simulink model "wheelmodsimscape"  (R2023a)
settings: Solver=ode23t  StartTime=0.0  StopTime=20  RelTol=1e-3
values from neighbouring files (symbols this model uses):
  angleT = 0    [rovervars.mat]    (also in varedit.m)
  mass = 1    [rovervars.mat]    (also in varedit.m)
  massRover = 50    [rovervars.mat]    (also in varedit.m)
  pwmVolt = 5    [rovervars.mat]    (also in varedit.m)
  radius = 0.1    [rovervars.mat]    (also in varedit.m)
  rotorInertia = 200    [rovervars.mat]    (also in varedit.m)
libraries: ee_lib x24, fl_lib x18, sdl_lib x13, nesl_utility x6, SignalEditorBlockLib x1
settings Model: Creator=MY DELL  LastModifiedBy=MY DELL

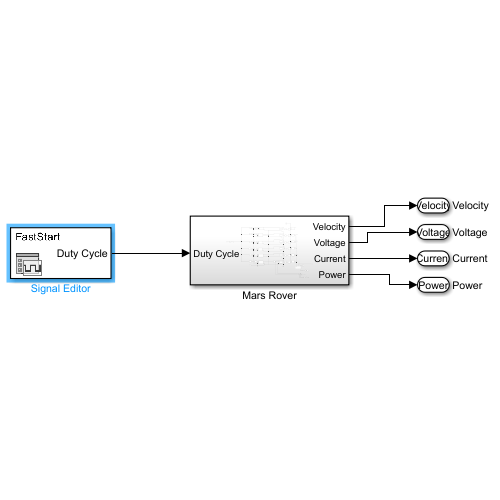
[thumbnail: Simulink's stored preview of the top-level diagram]
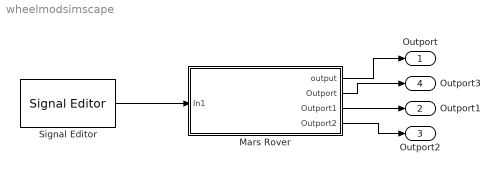
== system wheelmodsimscape ==
  Mars Rover : Subsystem
  Signal Editor : SignalEditorBlockLib/Signal Editor  FileName=signalscenario.mat  ActiveScenario=FastStart  ActiveSignal=Duty Cycle  IsBus=off  OutputBusObjectStr=Bus: BusObject  SampleTime=0  ZeroCross=off  OutputAfterFinalValue=Setting to zero  Unit=inherit  PreserveSignalName=on  ApplySigPropsToAllScenarios=on
  Outport : Outport  SignalName=Velocity
  Outport1 : Outport  Port=2  SignalName=Current
  Outport2 : Outport  Port=3  SignalName=Power
  Outport3 : Outport  Port=4  SignalName=Voltage
  wires:
  Signal Editor/1 -> Mars Rover/1(In1)
  Mars Rover/1(output) -> Outport/1
  Mars Rover/2(Outport) -> Outport3/1
  Mars Rover/3(Outport1) -> Outport1/1
  Mars Rover/4(Outport2) -> Outport2/1

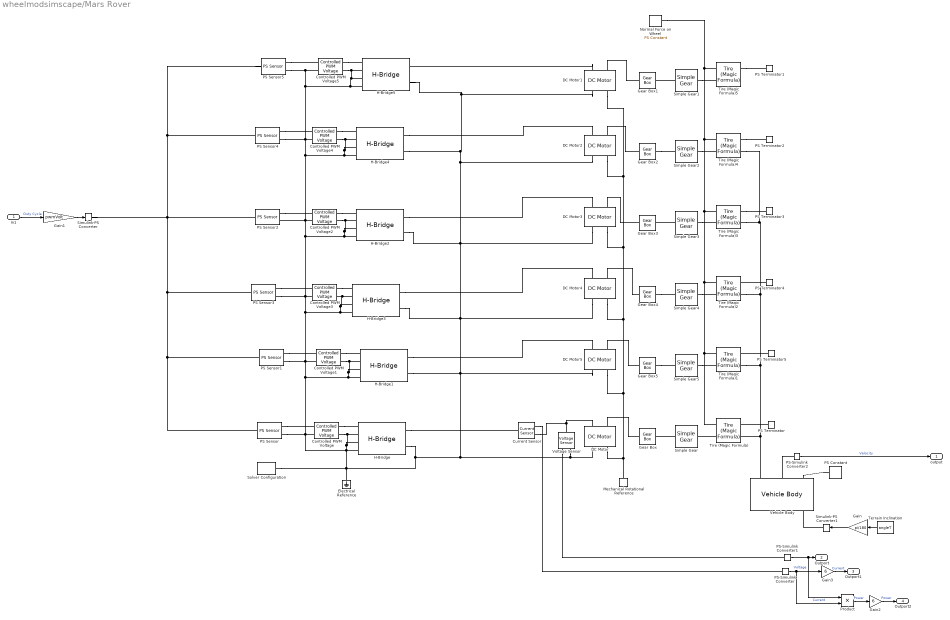
== system wheelmodsimscape/Mars Rover ==
  In1 : Inport
  Controlled PWM Voltage{,1..5} (6 alike) : ee_lib/Integrated Circuits/Controlled PWM Voltage  F=4000 Hz  TD=0 s  pulse_width_offset=0 s  pulse_min=0 s  pwm_or_av=ee.enum.pwm_or_av.averaged  event_type=ee.enum.ic.event.asynchronous  sample_time=1e-6 s  Vmin=0 V  Vmax=pwmVolt V  Vm=pwmVolt V  u_min=0  u_max=1
  Current Sensor : fl_lib/Electrical/Electrical Sensors/Current Sensor
  DC Motor{,1..5} (6 alike) : ee_lib/Electromechanical/Brushed Motors/DC Motor  field_option=ee.enum.field_option.pm  Rf=100 Ohm  Lf=1 H  Laf=0.15 H  If0=0 A  parameterization=ee.enum.dcparam_option.torque_speed  Ra=3.9 Ohm  La=inductance H  emf_or_torque=ee.enum.emf_or_torque.kv  Kv=0.072e-3 V/rpm  Ki=6.876e-4 N*m/A  T_stall=stallTorque N*m  w_max=noloadSpeed rpm  w_rated=15000 rpm  P_rated=0.08 W  V_rated=ratedVolt V  lam_param=ee.enum.lam_param.current  i_noload=noloadCurrent A  V_i_noload=ratedVolt V  J=rotorInertia cm^2*g  lam=0 N*m*s/rad  speed0=0 rpm  enable_fault_armature=simscape.enum.onoff.off  rev_faulted=1 / 3  G_faulted_armature=1e-5 S  fault_trigger_armature=ee.enum.faults.faultTrigger.temporal  t_fault_armature=1 s  max_permissible_current_armature=inf A  t_fail_on_current_armature=1 s  enable_fault_field=simscape.enum.onoff.off  G_faulted_field=1e-5 S  fault_trigger_field=ee.enum.faults.faultTrigger.temporal  t_fault_field=1 s  max_permissible_current_field=inf A  t_fail_on_current_field=1 s  fault_action=simscape.enum.assert.action.none  alpha=3.93e-3 1/K  Tmeas=25 degC  thermal_mass=100 J/K  initial_temperature=25 degC
  Electrical Reference : fl_lib/Electrical/Electrical Elements/Electrical Reference
  Gain : Gain  Gain=pi/180
  Gain1 : Gain  Gain=pwmVolt
  Gain2 : Gain  Gain=6
  Gain3 : Gain  Gain=6
  Gear Box{,1..5} (6 alike) : fl_lib/Mechanical/Mechanisms/Gear Box  ratio=100  t_in_specify=off  t_in_priority=None  t_in=0 N*m  t_in_nominal_specify=off  t_in_nominal_unit=N*m  t_in_nominal_value=1  t_out_specify=off  t_out_priority=None  t_out=0 N*m  t_out_nominal_specify=off  t_out_nominal_unit=N*m  t_out_nominal_value=1
  H-Bridge{,1..5} (6 alike) : ee_lib/Semiconductors & Converters/Converters/H-Bridge  supply_ports=ee.enum.supply_ports.hidesupply  pwm_or_av=ee.enum.pwm_or_av.averaged  regenerative_braking_mode=ee.enum.converters.regenerative_braking_mode.depends_on_rev  discontinuous=ee.enum.current_profile.continuous  freewheeling_mode=ee.enum.converters.freewheeling_mode.one_switch_one_diode  Rload=10 Ohm  Lload=1e-5 H  F=10 kHz  Venable=pwmVolt/2 V  Vmax=pwmVolt V  Vreverse=pwmVolt/2 V  Vbrake=pwmVolt/2 V  Vm=ratedVolt V  Ron=1e-6 Ohm  Don=0.05 Ohm  Goff=1e-6 S  Tmeas=298.15 K  Ron2=0.1 Ohm  Don2=0.05 Ohm  Tmeas2=398.15 K  thermal_mass=100 J/K  initial_temperature=298.15 K
  Mechanical Rotational Reference : fl_lib/Mechanical/Rotational Elements/Mechanical Rotational Reference
  Normal Force on Wheel : fl_lib/Physical Signals/Sources/PS Constant  constant=massRover*9.81/6 N
  PS Constant : fl_lib/Physical Signals/Sources/PS Constant  constant=windSpeed m/s
  PS Sensor{,1..5} (6 alike) : ee_lib/Sensors & Transducers/PS Sensor  op_type=1  A=1  B=0  Ymax=5  Ymin=0.01
      settings: InternalSimscapePortConfiguration="{\"Bottom\":[],\"Left\":[{\"id\":\"U\",\"label\":\"U\",\"type\":\"input\"}],\"Right\":[{\"id\":\"p\",\"label\":\"+\",\"type\":\"foundation.electrical.electrical\"},{\"id\":\"n\",\"label\":\"-\",\"type\":\"foundation.electrical.electrical\"}],\"Top\":[]}"
  PS Terminator{,1..5} (6 alike) : fl_lib/Physical Signals/Sinks/PS Terminator
  PS-Simulink Converter : nesl_utility/PS-Simulink Converter  PhysicalDomain=network_engine_domain  SubClassName=ps_output  LeftPortType=input  RightPortType=output  PseudoPeriodic=off  Frequencies=[]  VectorFormat=inherit  Unit=inherit  AffineConversion=off
  PS-Simulink Converter1 : nesl_utility/PS-Simulink Converter  PhysicalDomain=network_engine_domain  SubClassName=ps_output  LeftPortType=input  RightPortType=output  PseudoPeriodic=off  Frequencies=[]  VectorFormat=inherit  Unit=inherit  AffineConversion=off
  PS-Simulink Converter2 : nesl_utility/PS-Simulink Converter  PhysicalDomain=network_engine_domain  SubClassName=ps_output  LeftPortType=input  RightPortType=output  PseudoPeriodic=off  Frequencies=[]  VectorFormat=inherit  Unit=inherit  AffineConversion=off
  Product : Product
  Simple Gear{,1..5} (6 alike) : sdl_lib/Gears/Simple Gear  ratio=1  rotation_direction=sdl.enum.shaftOutputDirection.same  friction_model=sdl.enum.gear_efficiencies_load.constant  T_noload=0.1 N*m  T_nom=5 N*m  efficiency_nom=0.8  efficiency=0.8  temperature_TLU=[280, 300, 320] K  load_TLU=[1, 5, 10] N*m  efficiency_TLU=[.95, .9, .85]  efficiency_TLU2=[.85, .8, .75; .95, .9, .85; .85, .8, .7]  w_thr=0.01 rad/s  pwr_thr=0.001 W  enable_backlash=false  hardstop_model=simscape.enum.hardstop.smooth  backlash_distance=1e-3 mm  r_base=0.1 m  transition=1e-4 mm  backlash_stiffness=1e6 N/m  backlash_damping=1e3 N*s/m  coeff_rest=0.7  v_tol=0.001 m/s  f_tol=0.001 N  mu_visc=[0, 0] N*m*s/rad  enable_faults=simscape.enum.onoff.off  efficiency_fault=0.05  external_fault=simscape.enum.onoff.off  temporal_fault=simscape.enum.onoff.off  fault_time=5 s  fault_angles=pi / 12 rad  report_fault=simscape.enum.assert.action.none  thermal_mass=50 J/K  temperature_specify=off  temperature_priority=High  temperature=300 K  temperature_nominal_specify=off  temperature_nominal_unit=K  temperature_nominal_value=1  x_backlash_specify=off  x_backlash_priority=None  x_backlash=0 mm  x_backlash_nominal_specify=off  x_backlash_nominal_unit=mm  x_backlash_nominal_value=1  f_hardstop_specify=off  f_hardstop_priority=None  f_hardstop=0 N  f_hardstop_nominal_specify=off  f_hardstop_nominal_unit=N  f_hardstop_nominal_value=1  v_backlash_specify=off  v_backlash_priority=None  v_backlash=0 m/s  v_backlash_nominal_specify=off  v_backlash_nominal_unit=m/s  v_backlash_nominal_value=1
  Simulink-PS Converter : nesl_utility/Simulink-PS Converter  PhysicalDomain=network_engine_domain  SubClassName=ps_input  LeftPortType=input  RightPortType=output  PseudoPeriodic=off  Frequencies=[]  NoiseDistribution=none  NoiseParameters=[]  Unit=1  AffineConversion=off  FilteringAndDerivatives=provide  SimscapeFilterOrder=1  InputFilterTimeConstant=0.001  UdotUserProvided=0
  Simulink-PS Converter1 : nesl_utility/Simulink-PS Converter  PhysicalDomain=network_engine_domain  SubClassName=ps_input  LeftPortType=input  RightPortType=output  PseudoPeriodic=off  Frequencies=[]  NoiseDistribution=none  NoiseParameters=[]  Unit=1  AffineConversion=off  FilteringAndDerivatives=provide  SimscapeFilterOrder=1  InputFilterTimeConstant=0.001  UdotUserProvided=0
  Solver Configuration : nesl_utility/Solver Configuration  PhysicalDomain=network_engine_domain  SubClassName=solver  LeftPortType=input  RightPortType=generic  Tones=[]  Harmonics=[]  SimulateNoise=off  Profile=off  UseLocalSampling=off  EnableSwitchedLinearOptims=on  FrequencyDomain=off  UseCCode=off  RelTol=0.001  AbsTol=0.001  MinStep=1e-09  ToWorkspace=off  RevertToSquareIcSolve=off  NumHomotopyIterations=100  PhasorMode=off  PhasorModeNumHarmonics=1  ConsistencySolver=NEWTON_XTOL_AFTER_FTOL  IndexReductionMethod=DerivativeReplacement  DoDC=off  ResidualTolerance=1e-09  ConsistencyTolSource=GLOBAL  ConsistencyAbsTol=0.001  ConsistencyRelTol=0.001  ConsistencyTolFactor=0.001  UseLocalSolver=off  LocalSolverChoice=NE_BACKWARD_EULER_ADVANCER  ResolveIndetEquations=on  FunctionEvalNumThread=1  LocalSolverSampleTime=0.001  DoFixedCost=off  MaxNonlinIter=3  MaxModeIter=2  ComputeImpulses=off  ImpulseIterations=2  LinearAlgebra=auto  LinearAlgebraNumThread=0  EquationFormulation=NE_TIME_EF  DelaysMemoryBudget=1024  AutomaticFiltering=on  FilteringTimeConstant=0.001  PartitionStorageMethod=AS_NEEDED  PartitionMemoryBudget=1024  PartitionMethod=ROBUST
  Terrain Inclination : Constant  Value=angleT
  Tire (Magic Formula){,1..5} (6 alike) : sdl_lib/Tires & Vehicles/Tire (Magic Formula)  parameterization=sdl.enum.magic_tire_model.constant  F_z1=3000 N  F_x1=3500 N  kappa1=10  B_m=12  C_m=2.3  D_m=0.82  E_m=1  fz0=4000 N  p_Cx=1.685  p_Dx=[1.21, -.037]  p_Ex=[.344, .095, -.02, 0]  p_Kx=[21.51, -.163, .245]  p_Hx=[-.002, .002]  p_Vx=[0, 0]  rolling_radius_model=sdl.enum.RollingRadiusParameterization.Constant  r_e=radius m  r_0=0.3 m  breff=8.39  dreff=0.26  freff=0.074  q_re0=0.99  q_v1=0.008  longvl=17 m/s  cz=5e5 N/m  model_resistance=false  resistance_model=sdl.enum.rollingResistanceParameterization.constant  coeff=0.015  p_tire=250e3 Pa  alpha=-0.003  beta=0.97  coeff_a=84e-4  coeff_b=6.2e-4 s/m  coeff_c=1.6e-4 s^2/m^2  p_tire0=240e3 Pa  fz0_resistance=4000 N  vH0=16 m/s  q_Sy=[.0082, 0, .0014, .001, 0, 0, 1.08, -.5]  v_thr=0.001 m/s  enable_scaling_coefficients=false  lfzO=1  lcx=1  lmux=1  lex=1  lkx=1  lhx=1  lvx=1  lmy=1  model_compliance=sdl.enum.compliance.off  stiffness=1e6 N/m  damping=1000 N*s/m  model_inertia=sdl.enum.model_inertia.on  inertia=mass*radius^2 kg*m^2  initial_velocity=0 rad/s  vxlow=1 m/s  v_tr_thr=0.1 m/s  kpumin=-1.5  kpumax=1.5
  Vehicle Body : sdl_lib/Tires & Vehicles/Vehicle Body  mass=massRover kg  n_w=2  x_f=1.4 m  x_r=1.6 m  y_c=0.5 m  mass_var=simscape.enum.onoff.off  g=9.81 m/s^2  liftoff_warning=simscape.enum.onoff.off  area=area m^2  Cd=2.1  rho=1.18 kg/m^3  model_pitch=simscape.enum.onoff.off  inertia=4000 kg*m^2  suspension_model=sdl.enum.linearTLU.linear  k_f=1e4 N/m  b_f=1e4 N*s/m  k_r=1e4 N/m  b_r=1e4 N*s/m  k_f_TLU=[-2000, -1000, 0, 1000, 2000] N  x_f_TLU=[-.4, -.2, 0, .2, .4] m  b_f_TLU=[-200, -100, 0, 100, 200] N  v_f_TLU=[-4, -2, 0, 2, 4] m/s  k_r_TLU=[-2000, -1000, 0, 1000, 2000] N  x_r_TLU=[-.4, -.2, 0, .2, .4] m  b_r_TLU=[-200, -100, 0, 100, 200] N  v_r_TLU=[-4, -2, 0, 2, 4] m/s  interp_method=simscape.enum.interpolation.linear  extrap_method=simscape.enum.extrapolation.linear  model_hardstop=simscape.enum.onoff.off  upper_bound_f=.25 m  lower_bound_f=-.25 m  stop_k_f=1e6 N/m  stop_b_f=150 N*s/m  upper_bound_r=.25 m  lower_bound_r=-.25 m  stop_k_r=1e6 N/m  stop_b_r=150 N*s/m  initial_pitch=0 rad  initial_pitch_rate=0 rad/s  v_specify=off  v_priority=High  v=0 m/s  v_nominal_specify=off  v_nominal_unit=m/s  v_nominal_value=1
  Voltage Sensor : fl_lib/Electrical/Electrical Sensors/Voltage Sensor
  output : Outport
  Outport : Outport  Port=2
  Outport1 : Outport  Port=3
  Outport2 : Outport  Port=4
  wires:
  Gain/1 -> Simulink-PS Converter1/1
  Terrain Inclination/1 -> Gain/1
  Gain1/1 -> Simulink-PS Converter/1
  PS-Simulink Converter2/1 -> output/1  "Velocity"
  In1/1 -> Gain1/1  "Duty Cycle"
  PS-Simulink Converter1/1 -> Product/1, Outport/1  "Voltage"
  PS-Simulink Converter/1 -> Product/2, Gain3/1  "Current"
  Product/1 -> Gain2/1  "Power"
  Gain2/1 -> Outport2/1  "Power"
  Gain3/1 -> Outport1/1  "Current"
  connections:
  DC Motor/RConn2 -- DC Motor2/RConn2 -- DC Motor1/RConn2 -- DC Motor3/RConn2 -- DC Motor4/RConn2 -- DC Motor5/RConn2 -- Mechanical Rotational Reference/LConn1
  Vehicle Body/LConn2 -- PS-Simulink Converter2/LConn1
  Tire (Magic Formula)/LConn2 -- Simple Gear/RConn1
  PS Constant/RConn1 -- Vehicle Body/LConn3
  Vehicle Body/LConn1 -- Tire (Magic Formula)4/RConn2 -- Tire (Magic Formula)3/RConn2 -- Tire (Magic Formula)2/RConn2 -- Tire (Magic Formula)1/RConn2 -- Tire (Magic Formula)/RConn2
  PS Sensor/RConn1 -- Controlled PWM Voltage/LConn1
  Simple Gear/LConn1 -- Gear Box/RConn1
  Controlled PWM Voltage/RConn1 -- H-Bridge/LConn1
  Simulink-PS Converter1/RConn1 -- Vehicle Body/RConn3
  Normal Force on Wheel/RConn1 -- Tire (Magic Formula)5/LConn1 -- Tire (Magic Formula)4/LConn1 -- Tire (Magic Formula)3/LConn1 -- Tire (Magic Formula)2/LConn1 -- Tire (Magic Formula)1/LConn1 -- Tire (Magic Formula)/LConn1
  PS Terminator/LConn1 -- Tire (Magic Formula)/RConn1
  DC Motor/LConn2 -- Gear Box/LConn1
  Current Sensor/RConn2 -- Voltage Sensor/LConn1 -- DC Motor/LConn1
  Current Sensor/RConn1 -- PS-Simulink Converter/LConn1
  Voltage Sensor/RConn1 -- PS-Simulink Converter1/LConn1
  H-Bridge1/RConn1 -- DC Motor5/LConn1
  PS Sensor1/RConn1 -- Controlled PWM Voltage1/LConn1
  Controlled PWM Voltage1/RConn1 -- H-Bridge1/LConn1
  Simulink-PS Converter/RConn1 -- PS Sensor/LConn1 -- PS Sensor1/LConn1 -- PS Sensor3/LConn1 -- PS Sensor5/LConn1 -- PS Sensor4/LConn1 -- PS Sensor2/LConn1
  H-Bridge2/RConn1 -- DC Motor3/LConn1
  PS Sensor2/RConn1 -- Controlled PWM Voltage2/LConn1
  Controlled PWM Voltage2/RConn1 -- H-Bridge2/LConn1
  DC Motor3/RConn1 -- H-Bridge2/RConn2 -- H-Bridge3/RConn2 -- DC Motor4/RConn1 -- Solver Configuration/RConn1 -- Controlled PWM Voltage/RConn2 -- H-Bridge/LConn2 -- H-Bridge/LConn3 -- Controlled PWM Voltage/LConn2 -- PS Sensor/RConn2 -- H-Bridge1/LConn4 -- Controlled PWM Voltage1/RConn2 -- H-Bridge1/LConn2 -- H-Bridge1/LConn3 -- Controlled PWM Voltage1/LConn2 -- H-Bridge3/LConn4 -- Controlled PWM Voltage3/RConn2 -- H-Bridge3/LConn2 -- H-Bridge3/LConn3 -- PS Sensor3/RConn2 -- Controlled PWM Voltage3/LConn2 -- Controlled PWM Voltage4/LConn2 -- H-Bridge5/LConn3 -- Controlled PWM Voltage5/RConn2 -- H-Bridge5/LConn2 -- H-Bridge5/LConn4 -- PS Sensor5/RConn2 -- Controlled PWM Voltage5/LConn2 -- PS Sensor4/RConn2 -- H-Bridge4/LConn4 -- H-Bridge4/LConn3 -- Controlled PWM Voltage4/RConn2 -- H-Bridge4/LConn2 -- Controlled PWM Voltage2/LConn2 -- PS Sensor2/RConn2 -- H-Bridge2/LConn4 -- Controlled PWM Voltage2/RConn2 -- H-Bridge2/LConn2 -- H-Bridge2/LConn3 -- PS Sensor1/RConn2 -- H-Bridge/LConn4 -- Electrical Reference/LConn1 -- H-Bridge/RConn2 -- Voltage Sensor/RConn2 -- DC Motor/RConn1 -- DC Motor5/RConn1 -- H-Bridge1/RConn2 -- DC Motor2/RConn1 -- H-Bridge4/RConn2 -- H-Bridge5/RConn2 -- DC Motor1/RConn1
  H-Bridge3/RConn1 -- DC Motor4/LConn1
  PS Sensor3/RConn1 -- Controlled PWM Voltage3/LConn1
  Controlled PWM Voltage3/RConn1 -- H-Bridge3/LConn1
  Controlled PWM Voltage4/RConn1 -- H-Bridge4/LConn1
  PS Sensor4/RConn1 -- Controlled PWM Voltage4/LConn1
  H-Bridge4/RConn1 -- DC Motor2/LConn1
  Controlled PWM Voltage5/RConn1 -- H-Bridge5/LConn1
  PS Sensor5/RConn1 -- Controlled PWM Voltage5/LConn1
  DC Motor1/LConn1 -- H-Bridge5/RConn1
  DC Motor1/LConn2 -- Gear Box1/LConn1
  Simple Gear1/LConn1 -- Gear Box1/RConn1
  Simple Gear1/RConn1 -- Tire (Magic Formula)5/LConn2
  Simple Gear2/RConn1 -- Tire (Magic Formula)4/LConn2
  Gear Box2/RConn1 -- Simple Gear2/LConn1
  DC Motor2/LConn2 -- Gear Box2/LConn1
  DC Motor3/LConn2 -- Gear Box3/LConn1
  Simple Gear3/LConn1 -- Gear Box3/RConn1
  Simple Gear3/RConn1 -- Tire (Magic Formula)3/LConn2
  Simple Gear4/RConn1 -- Tire (Magic Formula)2/LConn2
  Gear Box4/RConn1 -- Simple Gear4/LConn1
  DC Motor4/LConn2 -- Gear Box4/LConn1
  Simple Gear5/RConn1 -- Tire (Magic Formula)1/LConn2
  Gear Box5/RConn1 -- Simple Gear5/LConn1
  DC Motor5/LConn2 -- Gear Box5/LConn1
  PS Terminator5/LConn1 -- Tire (Magic Formula)1/RConn1
  PS Terminator4/LConn1 -- Tire (Magic Formula)2/RConn1
  Tire (Magic Formula)3/RConn1 -- PS Terminator3/LConn1
  Tire (Magic Formula)4/RConn1 -- PS Terminator2/LConn1
  Tire (Magic Formula)5/RConn1 -- PS Terminator1/LConn1
  H-Bridge/RConn1 -- Current Sensor/LConn1
